simulink model "top_model"  (R2017a)
settings: Solver=FixedStepAuto  StartTime=0.0  StopTime=10.0  FixedStep=0.1  RelTol=1e-3
libraries: simulink x1
settings Model: Creator=The MathWorks, Inc.  LastModifiedBy=jdam
settings DataIOCC: LimitDataPoints=on
settings OptimizationCC: LifeSpan=inf
settings DebuggingCC: AllowSymbolicDim=off  SFUnexpectedBacktrackingDiag=warning  SFNoUnconditionalDefaultTransitionDiag=warning  SFExecutionAtInitializationDiag=none
settings ModelReferenceCC: PropagateSignalLabelsOutOfModel=off
settings GRTTargetCC: TargetLangStandard=C89/C90 (ANSI)
settings ConfigComp: CovMetricSettings=dw  CovHtmlReporting=on  CovSaveCumulativeToWorkspaceVar=on  CovSaveSingleToWorkspaceVar=on  CovExternalEMLEnable=off

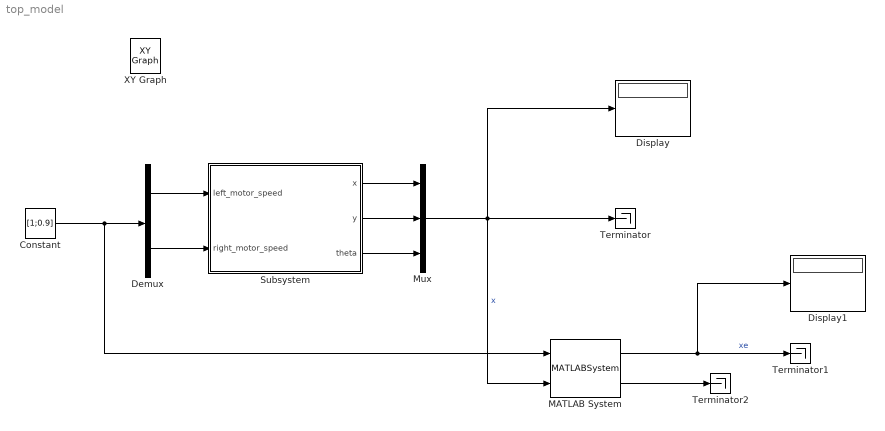
== system top_model ==
  Constant : Constant  Value=[1;0.9]  VectorParams1D=off
  Demux : Demux  Outputs=2
  Display : Display
  Display1 : Display
  MATLAB System : MATLABSystem  System=kalman  SimulateUsing=Code generation
      mask Type: kalman
      mask Display:
      | disp('kalman');
      | port_label('input',1,'u');
      | port_label('input',2,'z');
      | port_label('output',1,'xe');
      | port_label('output',2,'P');
  Mux : Mux  Inputs=3
  Subsystem : Subsystem
  Terminator : Terminator
  Terminator1 : Terminator
  Terminator2 : Terminator
  XY Graph : simulink/Sinks/XY Graph  IOType=viewer  xmin=-1  xmax=1  ymin=-1  ymax=1  st=-1
  wires:
  Demux/2 -> Subsystem/2(right_motor_speed)
  Demux/1 -> Subsystem/1(left_motor_speed)
  Subsystem/1(x) -> Mux/1
  Subsystem/2(y) -> Mux/2
  Constant/1 -> MATLAB System/1, Demux/1
  Subsystem/3(theta) -> Mux/3
  Mux/1 -> Display/1, Terminator/1, MATLAB System/2  "x"
  MATLAB System/1 -> Display1/1, Terminator1/1  "xe"
  MATLAB System/2 -> Terminator2/1

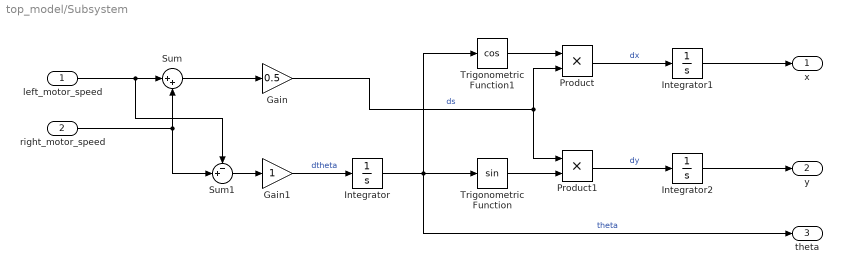
== system top_model/Subsystem ==
  left_motor_speed : Inport
  right_motor_speed : Inport  Port=2
  Gain : Gain  Gain=0.5
  Gain1 : Gain
  Integrator : Integrator
  Integrator1 : Integrator
  Integrator2 : Integrator
  Product : Product
  Product1 : Product
  Sum : Sum  Inputs=|++
  Sum1 : Sum  Inputs=-+|
  Trigonometric Function : Trigonometry
  Trigonometric Function1 : Trigonometry  Operator=cos
  x : Outport
  y : Outport  Port=2
  theta : Outport  Port=3
  wires:
  Integrator/1 -> theta/1, Trigonometric Function1/1, Trigonometric Function/1  "theta"
  Product/1 -> Integrator1/1  "dx"
  Sum1/1 -> Gain1/1
  Trigonometric Function/1 -> Product1/2
  Sum/1 -> Gain/1
  Gain/1 -> Product1/1, Product/2  "ds"
  Product1/1 -> Integrator2/1  "dy"
  Trigonometric Function1/1 -> Product/1
  Integrator1/1 -> x/1
  right_motor_speed/1 -> Sum1/2, Sum/2
  left_motor_speed/1 -> Sum1/1, Sum/1
  Gain1/1 -> Integrator/1  "dtheta"
  Integrator2/1 -> y/1
